simulink model "ClimateControl_with_SuperStep"  (R2018b)
settings: Solver=VariableStepAuto  StartTime=0.0  StopTime=10.0  RelTol=1e-3
libraries: simulink x2
settings Model: Creator=marwan  LastModifiedBy=marwan

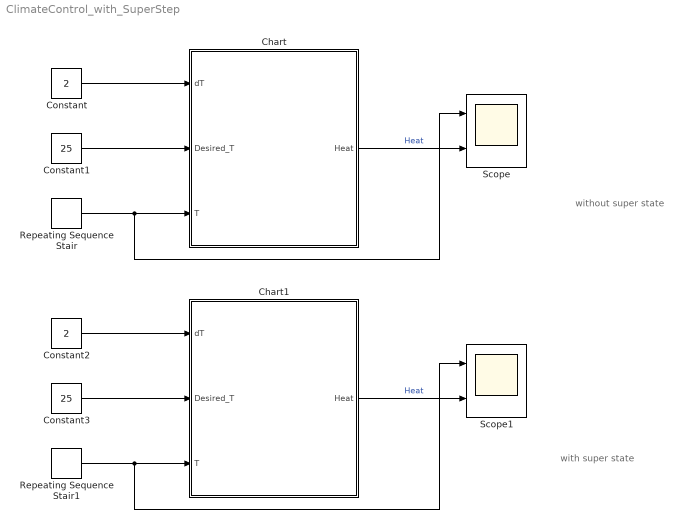
== system ClimateControl_with_SuperStep ==
  note: without super state
  note: with super state
  Chart : Stateflow chart  TreatAsAtomicUnit=on
  Chart1 : Stateflow chart  TreatAsAtomicUnit=on
  Constant : Constant  Value=2
  Constant1 : Constant  Value=25
  Constant2 : Constant  Value=2
  Constant3 : Constant  Value=25
  Repeating Sequence Stair : simulink/Sources/Repeating Sequence Stair  OutValues=a  tsamp=-1  OutMin=[]  OutMax=[]  OutDataTypeStr=double  OutputDataTypeScalingMode=double  OutDataType=fixdt(0,8)  ConRadixGroup=Best Precision: Vector-wise  OutScaling=2^-12
  Repeating Sequence Stair1 : simulink/Sources/Repeating Sequence Stair  OutValues=a  tsamp=-1  OutMin=[]  OutMax=[]  OutDataTypeStr=double  OutputDataTypeScalingMode=double  OutDataType=fixdt(0,8)  ConRadixGroup=Best Precision: Vector-wise  OutScaling=2^-12
  Scope : Scope  NumInputPorts=2
  Scope1 : Scope  NumInputPorts=2
  wires:
  Constant/1 -> Chart/1(dT)
  Constant1/1 -> Chart/2(Desired_T)
  Repeating Sequence Stair/1 -> Scope/1, Chart/3(T)
  Chart/1(Heat) -> Scope/2  "Heat"
  Chart1/1(Heat) -> Scope1/2  "Heat"
  Repeating Sequence Stair1/1 -> Chart1/3(T), Scope1/1
  Constant3/1 -> Chart1/2(Desired_T)
  Constant2/1 -> Chart1/1(dT)

== stateflow chart ClimateControl_with_SuperStep/Chart1 ==
  settings: enableNonTerminalStates=1
  state Off
    entry:
    Heat=0;
  state ColerOn
    entry:
    Heat=-1;
  state HeaterOn1
    entry:
    Heat=1;
  (default) -> (junction 26)
  (junction 26) -> Off
  ColerOn -> Off : [T<=Desired_T+dT]
  HeaterOn1 -> Off : [T>=Desired_T-dT]
  Off -> ColerOn [order 2] : [T>Desired_T+dT]
  Off -> HeaterOn1 [order 1] : [T<Desired_T-dT]
  data: dT input; Desired_T input; T input; Heat output

== stateflow chart ClimateControl_with_SuperStep/Chart ==
  state Off
    entry:
    Heat=0;
  state ColerOn
    entry:
    Heat=-1;
  state HeaterOn1
    entry:
    Heat=1;
  (default) -> (junction 26)
  (junction 26) -> ColerOn [order 2] : [[T>Desired_T+dT]]
  (junction 26) -> HeaterOn1 [order 1] : [T<Desired_T-dT]
  (junction 26) -> Off [order 3]
  ColerOn -> Off : [T<=Desired_T+dT]
  HeaterOn1 -> Off : [T>=Desired_T-dT]
  Off -> ColerOn [order 2] : [T>Desired_T+dT]
  Off -> HeaterOn1 [order 1] : [T<Desired_T-dT]
  data: dT input; Desired_T input; T input; Heat output
